simulink model "dialysisDemo"  (R2023a)
settings: Solver=VariableStepAuto  StartTime=0.0  StopTime=3600*4  RelTol=1e-3
undefined symbols (not defined in the file): out
libraries: SignalEditorBlockLib x3
settings Model: PacingRate=0.100000  Creator=alibacon  LastModifiedBy=tzhu
settings DebuggingCC: SubsystemReferenceDiagnosticForUnitTest=warning

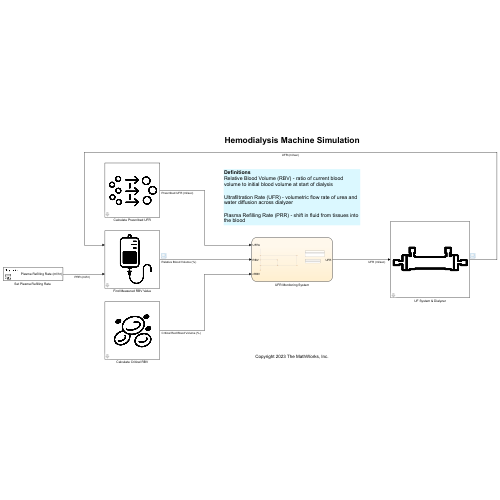
[thumbnail: Simulink's stored preview of the top-level diagram]
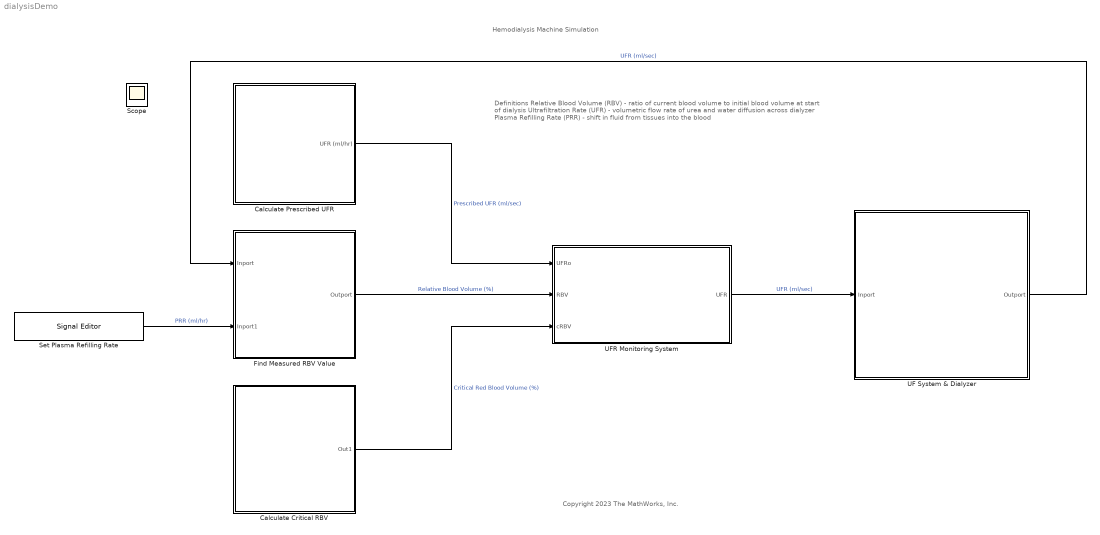
== system dialysisDemo ==
  note: Hemodialysis Machine Simulation
  note: Copyright 2023 The MathWorks, Inc.
  note: Definitions
      | Relative Blood Volume (RBV) - ratio of current blood volume to initial blood volume at start of dialysis
      |
      | Ultrafiltration Rate (UFR) - volumetric flow rate of urea and water diffusion across dialyzer
      |
      | Plasma Refilling Rate (PRR) - shift in fluid from tissues into the blood
  Calculate Critical RBV : Subsystem  mask{BPd=80, UF=2.6, DW=70.6, age=69, arrh=off, chf=off}
      mask prompts: BPd "Diastolic Blood Pressure (mmHg)"; UF "Target Ultrafiltration Volume (L)"; DW "Target Post-Dialysis Dry Weight (kg)"; age "Age (years)"; arrh "Prevalance of Arrythmia"; chf "Prevalance of Congestive Heart Failure Diagnosis"
      mask Display: image('medical-icons-red-blood-cell.png'); % Use "Edit Image" on toolstrip to change.
  Calculate Prescribed UFR : Subsystem  mask{predw=73.2, postdw=70.6, dtime=4}
      mask prompts: predw "Pre-Dialysis Weight (kg)"; postdw "Post-Dialysis Weight (kg)"; dtime "Dialysis Treatment Time (hr)"
      mask Display: image('medical-icons-ufr.png'); % Use "Edit Image" on toolstrip to change.
  Find Measured RBV Value : Subsystem  mask{BV0=3.774}
      mask prompts: BV0 "Initial Blood Volume (L)"
      mask Display: image('medical-icons-iv-bag.png'); % Use "Edit Image" on toolstrip to change.
  "Set Plasma Refilling Rate " : SignalEditorBlockLib/Signal Editor  FileName=dialysisDemo_PRR.mat  ActiveScenario=Scenario  ActiveSignal=Plasma Refilling Rate (ml/hr)  IsBus=off  OutputBusObjectStr=Bus: BusObject  SampleTime=0  Interpolate=off  ZeroCross=off  OutputAfterFinalValue=Setting to zero  Unit=inherit  PreserveSignalName=on  ApplySigPropsToAllScenarios=on
  UF System & Dialyzer : Subsystem  mask{DFR=30000}
      mask prompts: DFR "Dialysate Pump Flow Rate (ml/hr)"
      mask Display: image('medical-icons-dialyzer.png'); % Use "Edit Image" on toolstrip to change.
  UFR Monitoring System : Stateflow chart  TreatAsAtomicUnit=on
  Scope : Scope
  wires:
  "Set Plasma Refilling Rate "/1 -> Find Measured RBV Value/2(Inport1)  "PRR (ml/hr)"
  UFR Monitoring System/1(UFR) -> UF System & Dialyzer/1(Inport)  "UFR (ml/sec)"
  UF System & Dialyzer/1(Outport) -> Find Measured RBV Value/1(Inport)  "UFR (ml/sec)"
  Calculate Prescribed UFR/1(UFR (ml/hr)) -> UFR Monitoring System/1(UFRo)  "Prescribed UFR (ml/sec)"
  Find Measured RBV Value/1(Outport) -> UFR Monitoring System/2(RBV)  "Relative Blood Volume (%)"
  Calculate Critical RBV/1(Out1) -> UFR Monitoring System/3(cRBV)  "Critical Red Blood Volume (%)"

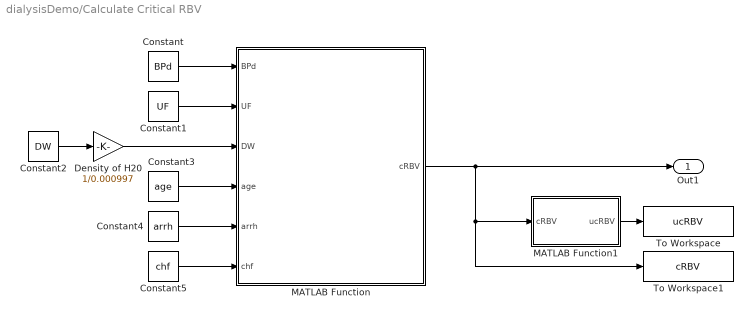
== system dialysisDemo/Calculate Critical RBV ==
  Constant : Constant  Value=BPd
  Constant1 : Constant  Value=UF
  Constant2 : Constant  Value=DW
  Constant3 : Constant  Value=age
  Constant4 : Constant  Value=arrh
  Constant5 : Constant  Value=chf
  Density of H20 : Gain  Gain=1/0.000997
  MATLAB Function : MATLAB Function  TreatAsAtomicUnit=on
  MATLAB Function1 : MATLAB Function  TreatAsAtomicUnit=on
  To Workspace : ToWorkspace  VariableName=ucRBV  SampleTime=-1
  To Workspace1 : ToWorkspace  VariableName=cRBV  SampleTime=-1
  Out1 : Outport
  wires:
  MATLAB Function/1(cRBV) -> To Workspace1/1, MATLAB Function1/1(cRBV), Out1/1
  Constant/1 -> MATLAB Function/1(BPd)
  Constant5/1 -> MATLAB Function/6(chf)
  Constant4/1 -> MATLAB Function/5(arrh)
  Constant3/1 -> MATLAB Function/4(age)
  Constant2/1 -> Density of H20/1
  Constant1/1 -> MATLAB Function/2(UF)
  Density of H20/1 -> MATLAB Function/3(DW)
  MATLAB Function1/1(ucRBV) -> To Workspace/1

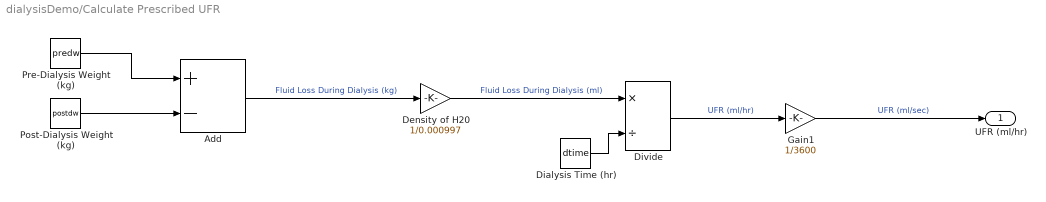
== system dialysisDemo/Calculate Prescribed UFR ==
  Add : Sum  Inputs=+-
  Density of H20 : Gain  Gain=1/0.000997
  Dialysis Time (hr) : Constant  Value=dtime
  Divide : Product  Inputs=*/
  Gain1 : Gain  Gain=1/3600
  Post-Dialysis Weight (kg) : Constant  Value=postdw
  Pre-Dialysis Weight (kg) : Constant  Value=predw
  UFR (ml/hr) : Outport
  wires:
  Add/1 -> Density of H20/1  "Fluid Loss During Dialysis (kg)"
  Divide/1 -> Gain1/1  "UFR (ml/hr)"
  Pre-Dialysis Weight (kg)/1 -> Add/1
  Density of H20/1 -> Divide/1  "Fluid Loss During Dialysis (ml)"
  Post-Dialysis Weight (kg)/1 -> Add/2
  Dialysis Time (hr)/1 -> Divide/2
  Gain1/1 -> UFR (ml/hr)/1  "UFR (ml/sec)"

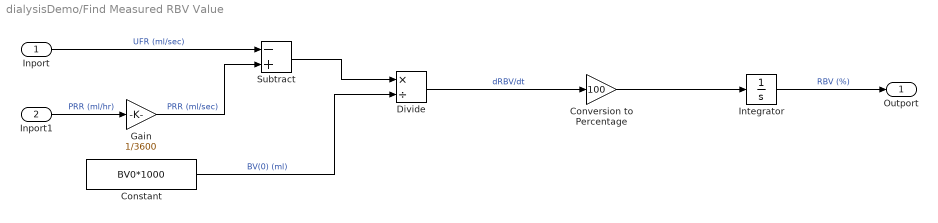
== system dialysisDemo/Find Measured RBV Value ==
  Inport : Inport
  Inport1 : Inport  Port=2
  Constant : Constant  Value=BV0*1000
  Conversion to Percentage : Gain  Gain=100
  Divide : Product  Inputs=*/
  Gain : Gain  Gain=1/3600
  Integrator : Integrator  InitialCondition=100
  Subtract : Sum  Inputs=-+
  Outport : Outport
  wires:
  Integrator/1 -> Outport/1  "RBV (%)"
  Divide/1 -> Conversion to Percentage/1  "dRBV/dt"
  Subtract/1 -> Divide/1
  Constant/1 -> Divide/2  "BV(0) (ml)"
  Inport/1 -> Subtract/1  "UFR (ml/sec)"
  Inport1/1 -> Gain/1  "PRR (ml/hr)"
  Conversion to Percentage/1 -> Integrator/1
  Gain/1 -> Subtract/2  "PRR (ml/sec)"

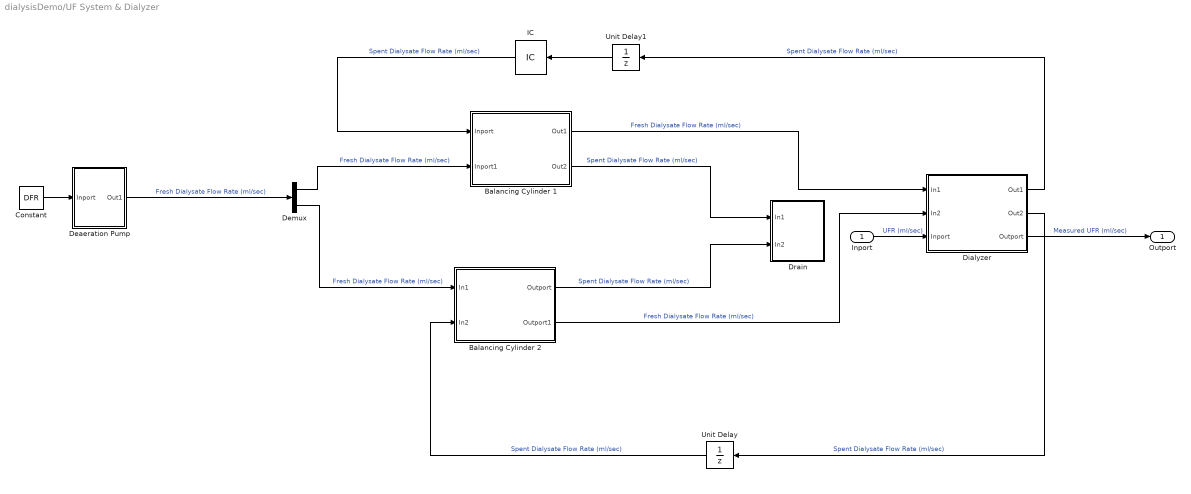
== system dialysisDemo/UF System & Dialyzer ==
  Inport : Inport
  Balancing Cylinder 1 : Subsystem
  Balancing Cylinder 2 : Subsystem
  Constant : Constant  Value=DFR
  Deaeration Pump : Subsystem
  Demux : Demux  Outputs=2
  Dialyzer : Subsystem
  Drain : Subsystem
  IC : InitialCondition  Value=DFR
  Unit Delay : UnitDelay  SampleTime=-1  HasFrameUpgradeWarning=on
  Unit Delay1 : UnitDelay  SampleTime=-1  HasFrameUpgradeWarning=on
  Outport : Outport
  wires:
  IC/1 -> Balancing Cylinder 1/1(Inport)  "Spent Dialysate Flow Rate (ml/sec)"
  Balancing Cylinder 2/2(Outport1) -> Dialyzer/2(In2)  "Fresh Dialysate Flow Rate (ml/sec)"
  Deaeration Pump/1(Out1) -> Demux/1  "Fresh Dialysate Flow Rate (ml/sec)"
  Dialyzer/1(Out1) -> Unit Delay1/1  "Spent Dialysate Flow Rate (ml/sec)"
  Demux/2 -> Balancing Cylinder 2/1(In1)  "Fresh Dialysate Flow Rate (ml/sec)"
  Unit Delay1/1 -> IC/1
  Unit Delay/1 -> Balancing Cylinder 2/2(In2)  "Spent Dialysate Flow Rate (ml/sec)"
  Balancing Cylinder 1/1(Out1) -> Dialyzer/1(In1)  "Fresh Dialysate Flow Rate (ml/sec)"
  Balancing Cylinder 2/1(Outport) -> Drain/2(In2)  "Spent Dialysate Flow Rate (ml/sec)"
  Demux/1 -> Balancing Cylinder 1/2(Inport1)  "Fresh Dialysate Flow Rate (ml/sec)"
  Balancing Cylinder 1/2(Out2) -> Drain/1(In1)  "Spent Dialysate Flow Rate (ml/sec)"
  Constant/1 -> Deaeration Pump/1(Inport)
  Dialyzer/2(Out2) -> Unit Delay/1  "Spent Dialysate Flow Rate (ml/sec)"
  Inport/1 -> Dialyzer/3(Inport)  "UFR (ml/sec)"
  Dialyzer/3(Outport) -> Outport/1  "Measured UFR (ml/sec)"

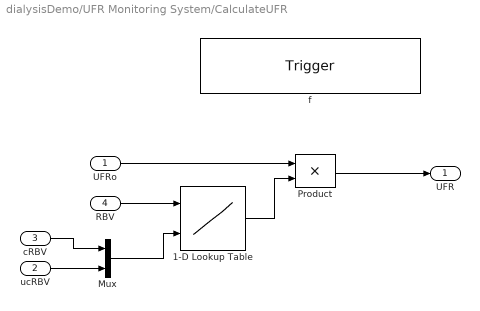
== system dialysisDemo/UFR Monitoring System/CalculateUFR ==
  UFRo : Inport  OutDataTypeStr=double  PortDimensions=1
  ucRBV : Inport  Port=2  OutDataTypeStr=double  PortDimensions=1
  cRBV : Inport  Port=3  OutDataTypeStr=double  PortDimensions=1
  RBV : Inport  Port=4  OutDataTypeStr=double  PortDimensions=1
  f : TriggerPort  TriggerType=function-call  VariantControl=(inherit)
      settings: CopyFcn=Stateflow.SLINSF.SimulinkMan.removeBlockPreDeleteFcn  PreDeleteFcn=Stateflow.SLINSF.SimulinkMan.unsafePredeleteFcn
  1-D Lookup Table : Lookup_n-D  NumberOfTableDimensions=1  BreakpointsForDimension1Source=Input port  BreakpointsForDimension1=[out.cRBV out.ucRBV]  Table=[0 1]  InternalRulePriority=Speed  RndMeth=Simplest
      settings: InputPortMap=u0,p5
  Mux : Mux  Inputs=2
  Product : Product
  UFR : Outport
  wires:
  RBV/1 -> 1-D Lookup Table/1
  cRBV/1 -> Mux/1
  UFRo/1 -> Product/1
  Mux/1 -> 1-D Lookup Table/2
  ucRBV/1 -> Mux/2
  1-D Lookup Table/1 -> Product/2
  Product/1 -> UFR/1

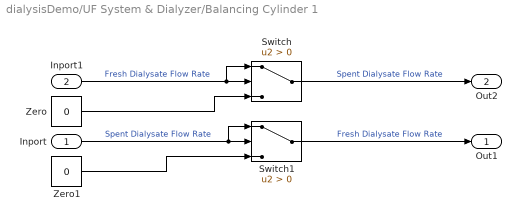
== system dialysisDemo/UF System & Dialyzer/Balancing Cylinder 1 ==
  Inport : Inport
  Inport1 : Inport  Port=2
  Switch : Switch  Criteria=u2 > Threshold  SaturateOnIntegerOverflow=off  InputSameDT=off
  Switch1 : Switch  Criteria=u2 > Threshold  SaturateOnIntegerOverflow=off  InputSameDT=off
  Zero : Constant  Value=0  OutDataTypeStr=Inherit: Inherit via back propagation
  Zero1 : Constant  Value=0  OutDataTypeStr=Inherit: Inherit via back propagation
  Out1 : Outport
  Out2 : Outport  Port=2
  wires:
  Inport1/1 -> Switch/1, Switch/2  "Fresh Dialysate Flow Rate"
  Inport/1 -> Switch1/1, Switch1/2  "Spent Dialysate Flow Rate"
  Switch1/1 -> Out1/1  "Fresh Dialysate Flow Rate"
  Switch/1 -> Out2/1  "Spent Dialysate Flow Rate"
  Zero/1 -> Switch/3
  Zero1/1 -> Switch1/3

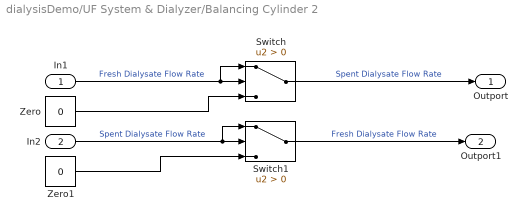
== system dialysisDemo/UF System & Dialyzer/Balancing Cylinder 2 ==
  In1 : Inport
  In2 : Inport  Port=2
  Switch : Switch  Criteria=u2 > Threshold  SaturateOnIntegerOverflow=off  InputSameDT=off
  Switch1 : Switch  Criteria=u2 > Threshold  SaturateOnIntegerOverflow=off  InputSameDT=off
  Zero : Constant  Value=0  OutDataTypeStr=Inherit: Inherit via back propagation
  Zero1 : Constant  Value=0  OutDataTypeStr=Inherit: Inherit via back propagation
  Outport : Outport
  Outport1 : Outport  Port=2
  wires:
  In1/1 -> Switch/1, Switch/2  "Fresh Dialysate Flow Rate"
  In2/1 -> Switch1/1, Switch1/2  "Spent Dialysate Flow Rate"
  Switch1/1 -> Outport1/1  "Fresh Dialysate Flow Rate"
  Switch/1 -> Outport/1  "Spent Dialysate Flow Rate"
  Zero/1 -> Switch/3
  Zero1/1 -> Switch1/3

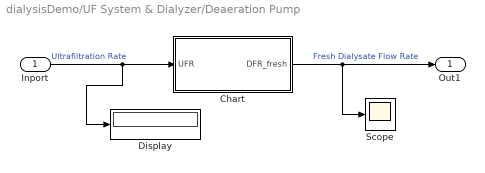
== system dialysisDemo/UF System & Dialyzer/Deaeration Pump ==
  Inport : Inport
  Chart : Stateflow chart  TreatAsAtomicUnit=on
  Display : Display
  Scope : Scope
  Out1 : Outport
  wires:
  Inport/1 -> Display/1, Chart/1(UFR)  "Ultrafiltration Rate"
  Chart/1(DFR_fresh) -> Scope/1, Out1/1  "Fresh Dialysate Flow Rate"

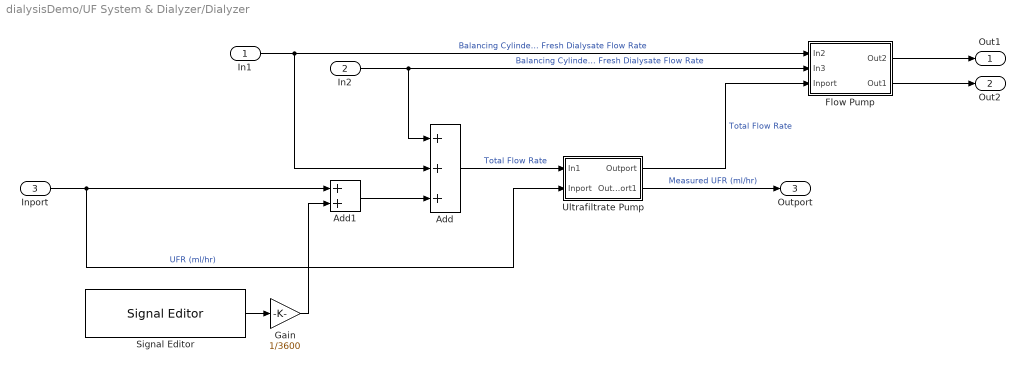
== system dialysisDemo/UF System & Dialyzer/Dialyzer ==
  In1 : Inport
  In2 : Inport  Port=2
  Inport : Inport  Port=3
  Add : Sum  Inputs=+++
  Add1 : Sum
  Flow Pump : Subsystem
  Gain : Gain  Gain=1/3600
  Signal Editor : SignalEditorBlockLib/Signal Editor  FileName=dialysisDemo_noise.mat  ActiveScenario=UltrafiltrationRate  ActiveSignal=UFR Noise (ml/hr)  IsBus=off  OutputBusObjectStr=Bus: BusObject  SampleTime=0  Interpolate=off  ZeroCross=off  OutputAfterFinalValue=Setting to zero  Unit=inherit  PreserveSignalName=on  ApplySigPropsToAllScenarios=on
  Ultrafiltrate Pump : Subsystem
  Out1 : Outport
  Out2 : Outport  Port=2
  Outport : Outport  Port=3
  wires:
  In2/1 -> Add/1, Flow Pump/2(In3)  "Balancing Cylinder 2 Fresh Dialysate Flow Rate"
  In1/1 -> Add/2, Flow Pump/1(In2)  "Balancing Cylinder 1 Fresh Dialysate Flow Rate"
  Add/1 -> Ultrafiltrate Pump/1(In1)  "Total Flow Rate"
  Flow Pump/2(Out1) -> Out2/1
  Flow Pump/1(Out2) -> Out1/1
  Ultrafiltrate Pump/1(Outport) -> Flow Pump/3(Inport)  "Total Flow Rate"
  Inport/1 -> Add1/1, Ultrafiltrate Pump/2(Inport)  "UFR (ml/hr)"
  Ultrafiltrate Pump/2(Outport1) -> Outport/1  "Measured UFR (ml/hr)"
  Add1/1 -> Add/3
  Signal Editor/1 -> Gain/1
  Gain/1 -> Add1/2

== system dialysisDemo/UF System & Dialyzer/Drain ==
  In1 : Inport
  In2 : Inport  Port=2
  Terminator : Terminator
  Terminator1 : Terminator
  wires:
  In1/1 -> Terminator/1
  In2/1 -> Terminator1/1

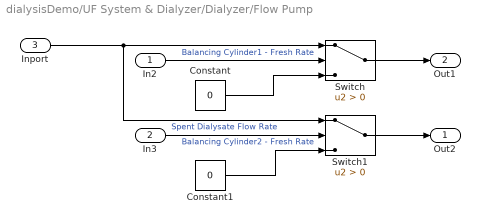
== system dialysisDemo/UF System & Dialyzer/Dialyzer/Flow Pump ==
  In2 : Inport
  In3 : Inport  Port=2
  Inport : Inport  Port=3
  Constant : Constant  Value=0  SampleTime=-1
  Constant1 : Constant  Value=0  SampleTime=-1
  Switch : Switch  Criteria=u2 > Threshold  SaturateOnIntegerOverflow=off  InputSameDT=off
  Switch1 : Switch  Criteria=u2 > Threshold  SaturateOnIntegerOverflow=off  InputSameDT=off
  Out2 : Outport
  Out1 : Outport  Port=2
  wires:
  Inport/1 -> Switch/1, Switch1/1  "Spent Dialysate Flow Rate"
  In2/1 -> Switch/2  "Balancing Cylinder1 - Fresh Rate"
  Switch/1 -> Out1/1
  Constant/1 -> Switch/3
  In3/1 -> Switch1/2  "Balancing Cylinder2 - Fresh Rate"
  Switch1/1 -> Out2/1
  Constant1/1 -> Switch1/3

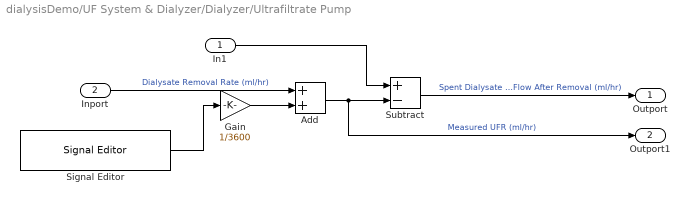
== system dialysisDemo/UF System & Dialyzer/Dialyzer/Ultrafiltrate Pump ==
  In1 : Inport
  Inport : Inport  Port=2
  Add : Sum
  Gain : Gain  Gain=1/3600
  Signal Editor : SignalEditorBlockLib/Signal Editor  FileName=dialysisDemo_noise.mat  ActiveScenario=UltrafiltratePump  ActiveSignal=UF Pump Noise (ml/hr)  IsBus=off  OutputBusObjectStr=Bus: BusObject  SampleTime=0  Interpolate=off  ZeroCross=off  OutputAfterFinalValue=Setting to zero  Unit=inherit  PreserveSignalName=on  ApplySigPropsToAllScenarios=on
  Subtract : Sum  Inputs=+-
  Outport : Outport
  Outport1 : Outport  Port=2
  wires:
  In1/1 -> Subtract/1
  Subtract/1 -> Outport/1  "Spent Dialysate Flow After Removal (ml/hr)"
  Inport/1 -> Add/1  "Dialysate Removal Rate (ml/hr)"
  Add/1 -> Outport1/1, Subtract/2  "Measured UFR (ml/hr)"
  Signal Editor/1 -> Gain/1
  Gain/1 -> Add/2

== matlab function dialysisDemo/Calculate Critical RBV/MATLAB Function ==
  data: BPd input; cRBV output; UF input; DW input; age input; arrh input; chf input
function cRBV = calculate_cRBV(BPd, UF, DW, age, arrh, chf)
% BPd - diastolic blood pressure at t=0 (mmHg)
% UF -  (l)
% DW - target dry weight post-dialysis (l)
% age - age in years (yrs)
% arrh - prevalence of arrythmia (0=absent; 1=existent)
% chf - prevalence of congestive heart failure diagnosis (0=absent; 1=existent)

cRBV = 97.8 - 0.08*BPd - (UF/DW) + 0.05*age + 1.5*arrh + 0.2*chf;

== stateflow chart dialysisDemo/UF System & Dialyzer/Deaeration Pump/Chart ==
  state FillCylinder2
    entry: DFR_fresh = [UFR, 0];
    during: DFR_fresh = [UFR, 0];
  state FillCylinder1
    entry: DFR_fresh = [0, UFR];
    during: DFR_fresh = [0, UFR];
  (default) -> FillCylinder1
  FillCylinder2 -> FillCylinder1 : after(30*3600/UFR, sec)
  FillCylinder1 -> FillCylinder2 : after(30*3600/UFR, sec)
  data: UFR input; DFR_fresh output

== matlab function dialysisDemo/Calculate Critical RBV/MATLAB Function1 ==
  data: cRBV input; ucRBV output
function ucRBV = fcn(cRBV)
% Calculate the upper threshold for cRBV where UFR begins to decrease
ucRBV = (100 - cRBV) / 2 + cRBV;

== stateflow chart dialysisDemo/UFR Monitoring System ==
  state UFR = CalculateUFR(UFRo,ucRBV,cRBV,RBV) [function]
  (default) -> (junction 55) : {
      | ucRBV = CalculateUcRBV(cRBV)
      | }
  (junction 55) -> (junction 56) [order 1] : [RBV<=cRBV]
  (junction 55) -> (junction 57) [order 2]
  (junction 56) -> (junction 61) : {UFR=0;}
  (junction 57) -> (junction 58) [order 1] : [(cRBV < RBV) && (RBV < ucRBV)]
  (junction 57) -> (junction 59) [order 2] : {UFR = UFRo;}
  (junction 58) -> (junction 60) : {UFR = CalculateUFR(UFRo,ucRBV,cRBV,RBV);}
  (junction 60) -> (junction 59)
  (junction 61) -> (junction 60)
  (junction 59) -> (junction 62)
  data: UFRo function_input double size=1; ucRBV function_input double size=1; cRBV function_input double size=1; RBV function_input double size=1; UFR function_output; cRBVInput function_input; ucRBV function_output; UFR output size=1; UFRo input size=1; RBV input size=1; cRBV input size=1; ucRBV local
  function ucRBV = CalculateUcRBV(cRBVInput):
    | function ucRBV = CalculateUcRBV(cRBVInput)
    | % Calculate the upper threshold for cRBV where UFR begins to decrease
    | ucRBV = (100 - cRBVInput) / 2 + cRBVInput;
